simulink model "controle_01"  (R2014b)
settings: Solver=ode45  StartTime=0.0  StopTime=t_run  RelTol=1e-3
values from neighbouring files (symbols this model uses):
  den_G = G.den{:}    [sim_02.m]
  num_G = G.num{:}    [sim_02.m]
  t_step = 1    [sim_02.m]
undefined symbols (not defined in the file or in its folder): den_C, num_C
settings Model: Creator=PC  LastModifiedBy=PC

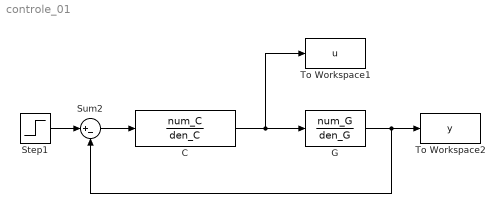
== system controle_01 ==
  C : TransferFcn  Numerator=num_C  Denominator=den_C
  G : TransferFcn  Numerator=num_G  Denominator=den_G
  Step1 : Step  Time=t_step
  Sum2 : Sum  Inputs=|+-
  To Workspace1 : ToWorkspace  VariableName=u  SampleTime=-1
  To Workspace2 : ToWorkspace  VariableName=y  SampleTime=-1
  wires:
  Sum2/1 -> C/1
  G/1 -> To Workspace2/1, Sum2/2
  C/1 -> To Workspace1/1, G/1
  Step1/1 -> Sum2/1
